simulink model "tank1_hydraulic_model_old"  (R2025a)
settings: Solver=ode45  StartTime=0.0  StopTime=1200  RelTol=1e-3
settings Model: Creator=Vanshish_PC  LastModifiedBy=Vanshish_PC

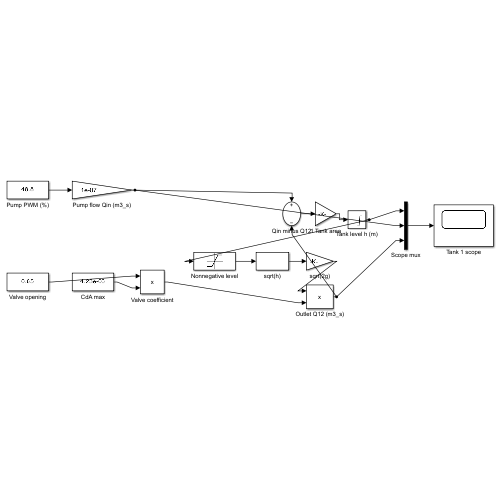
[thumbnail: Simulink's stored preview of the top-level diagram]
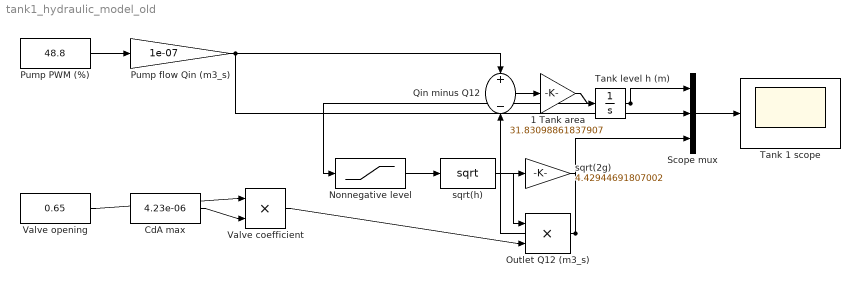
== system tank1_hydraulic_model_old ==
  1 Tank area : Gain  Gain=31.83098861837907
  CdA max : Constant  Value=4.23e-06
  Nonnegative level : Saturate  UpperLimit=0.3  LowerLimit=0
  Outlet Q12 (m3_s) : Product  Inputs=**
  Pump PWM (%) : Constant  Value=48.8
  Pump flow Qin (m3_s) : Gain  Gain=1e-07
  Qin minus Q12 : Sum  Inputs=+-
  Scope mux : Mux  Inputs=3
  Tank 1 scope : Scope
  Tank level h (m) : Integrator  InitialCondition=0.16  LimitOutput=on  UpperSaturationLimit=0.3  LowerSaturationLimit=0
  Valve coefficient : Product  Inputs=**
  Valve opening : Constant  Value=0.65
  sqrt(2g) : Gain  Gain=4.42944691807002
  sqrt(h) : Math  Operator=sqrt
  wires:
  Pump PWM (%)/1 -> Pump flow Qin (m3_s)/1
  Pump flow Qin (m3_s)/1 -> Qin minus Q12/1, Scope mux/2
  Valve opening/1 -> Valve coefficient/1
  CdA max/1 -> Valve coefficient/2
  Tank level h (m)/1 -> Nonnegative level/1, Scope mux/1
  Nonnegative level/1 -> sqrt(h)/1
  sqrt(h)/1 -> sqrt(2g)/1
  sqrt(2g)/1 -> Outlet Q12 (m3_s)/1
  Valve coefficient/1 -> Outlet Q12 (m3_s)/2
  Outlet Q12 (m3_s)/1 -> Qin minus Q12/2, Scope mux/3
  Qin minus Q12/1 -> 1 Tank area/1
  1 Tank area/1 -> Tank level h (m)/1
  Scope mux/1 -> Tank 1 scope/1
